simulink subsystem "PvtSubSys_LSM"  (R2020b)
settings: Solver=VariableStepAuto  StartTime=0.0  StopTime=10.0  RelTol=1e-3
values from neighbouring files (symbols this model uses):
  P_LSM_ALC_Enable = 0.0    [LSM_Parameter.sldd]
  P_LSM_DOP_C0_EN_Limit = 0.8    [LSM_Parameter.sldd]
  P_LSM_DOP_C0_out_Limit = 2.0    [LSM_Parameter.sldd]
  P_LSM_DOP_C1_EN_Limit : value not decoded    [LSM_Parameter.sldd]
  P_LSM_DOP_C1_out_Limit : value not decoded    [LSM_Parameter.sldd]
  P_LSM_DOP_C1AndC2_Lim_X : value not decoded    [LSM_Parameter.sldd]
  P_LSM_DOP_C2_EN_Limit : value not decoded    [LSM_Parameter.sldd]
  P_LSM_DOP_C2_out_Limit : value not decoded    [LSM_Parameter.sldd]
  P_LSM_DOP_In_Pre2Dop_Dis = 1.0    [LSM_Parameter.sldd]
  P_LSM_DOP_Out_Pre2Dop_Dis = 2.0    [LSM_Parameter.sldd]
  P_LSM_DOP_PreDis_X : value not decoded    [LSM_Parameter.sldd]
  P_LSM_DOP_PreDis_Y : value not decoded    [LSM_Parameter.sldd]
  P_LSM_DOPValid_CheckTime = 0.06    [LSM_Parameter.sldd]
  P_LSM_DoubleLine_Curr2Cent_Dislimit = 0.5    [LSM_Parameter.sldd]
  P_LSM_DoubleLine_Dop2Cent_Dislimit = 0.5    [LSM_Parameter.sldd]
  P_LSM_DoubleLine_DOPOut_C1 : value not decoded    [LSM_Parameter.sldd]
  P_LSM_DoubleLine_Pre2Cent_Dislimit = 1.0    [LSM_Parameter.sldd]
  P_LSM_IFV2CenterAxis = 0.0    [LSM_Parameter.sldd]
  P_LSM_IFV2RearAxis = 0.0    [LSM_Parameter.sldd]
  P_LSM_LineSTD_Limit = 0.15    [LSM_Parameter.sldd]
  P_LSM_NOH_Switch = 0.0    [LSM_Parameter.sldd]
  P_LSM_Pre_t = 0.0    [LSM_Parameter.sldd]
  P_LSM_SingleLine_Cent2Edge_Dislimit = 100.0    [LSM_Parameter.sldd]
  P_LSM_SingleLine_Curr2Cent_Dislimit = 0.2    [LSM_Parameter.sldd]
  P_LSM_SingleLine_Dop2Cent_Dislimit = 0.2    [LSM_Parameter.sldd]
  P_LSM_SingleLine_DOPOut_C1 : value not decoded    [LSM_Parameter.sldd]
  P_LSM_SingleLine_Pre2Cent_Dislimit = 0.5    [LSM_Parameter.sldd]
undefined symbols (not defined in the file or in its folder): P_LSM_LineWijCal_C12, P_LSM_LineWijCal_C13, P_LSM_PosLineLcFac
libraries: simulink x92, TrueDurationTime x2
(part 5 of 9)

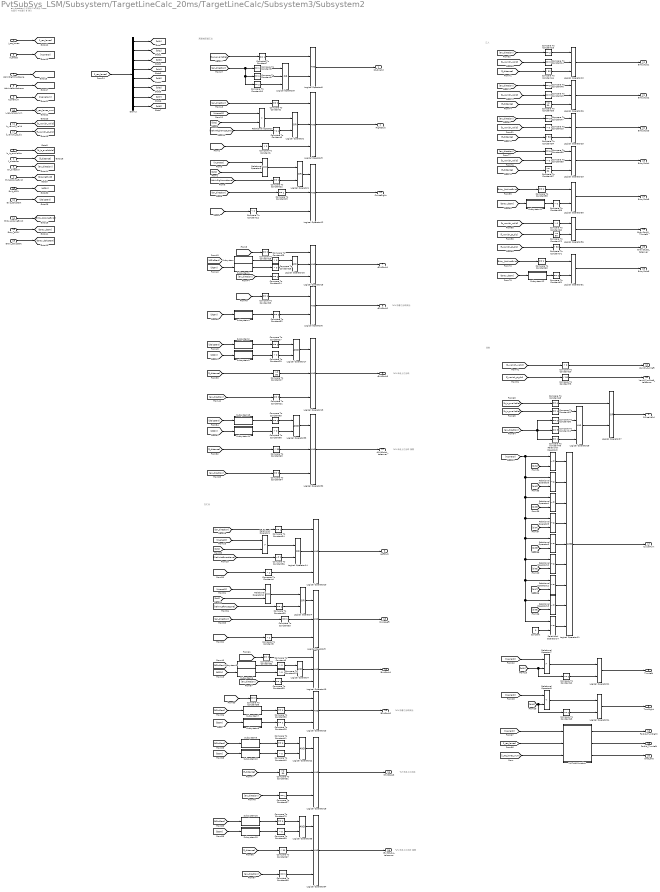
== system PvtSubSys_LSM/Subsystem/TargetLineCalc_20ms/TargetLineCalc/Subsystem3/Subsystem2 ==
  note: 左汇出
  note: 巡航
  note: 汇入
  note: %%未走上汇出线
  note: %%沿着汇出线驶出
  note: %%未走上汇出线
  note: en_direction
      | 1 左驶出
      | 2 右驶出
      | 3 左直行
      | 4 右直行
      | 5 驶入
  note: %%沿着汇出线驶出
  note: 高速或匝道汇出
  note: %%未走上汇出线,接管
  note: %%未走上汇出线,接管
  Exit_bIsLineExist : Inport
  f_distance : Inport  Port=2
  b_is_available : Inport  Port=3
  i_rec_lanes : Inport  Port=4
  nLaneID : Inport  Port=5
  en_direction : Inport  Port=6
  VehInRightmostLane : Inport  Port=7  OutDataTypeStr=boolean
  VehInLeftmostLane : Inport  Port=8  OutDataTypeStr=boolean
  nLaneNum : Inport  Port=9
  i_rec_lanes_num : Inport  Port=10
  " b_vanish_valid" : Inport  Port=11
  " Exit_dDisStart" : Inport  Port=12
  Exit_dC0V : Inport  Port=13
  Entry_bIsLineExist : Inport  Port=14
  Entry_dDisStart : Inport  Port=15
  Entry_dC0V : Inport  Port=16
  " f_vanish_pt_dis " : Inport  Port=17
  Compare To Constant{1,4..5,12} (4 alike) : simulink/Logic and Bit Operations/Compare To Constant  relop=<  const=2  OutDataTypeStr=boolean
  Compare To Constant{10,16,46..47,56} (5 alike) : simulink/Logic and Bit Operations/Compare To Constant  relop===  const=5  OutDataTypeStr=boolean
  Compare To Constant11 : simulink/Logic and Bit Operations/Compare To Constant  relop===  const=3  OutDataTypeStr=boolean
  Compare To Constant{6,13,15,20,25..26,29,40,55,59,62,66,69} (13 alike) : simulink/Logic and Bit Operations/Compare To Constant  relop=>  const=0  OutDataTypeStr=boolean
  Compare To Constant{14,27..28,30,41,45,48,50,52,61,65,70} (12 alike) : simulink/Logic and Bit Operations/Compare To Constant  relop===  const=0  OutDataTypeStr=boolean
  Compare To Constant17 : simulink/Logic and Bit Operations/Compare To Constant  relop=>=  const=50  OutDataTypeStr=boolean
  Compare To Constant{2,9,18..19,21,23..24,32,38,58,60,64} (12 alike) : simulink/Logic and Bit Operations/Compare To Constant  relop===  const=2  OutDataTypeStr=boolean
  Compare To Constant{7..8,22,33..35,37,39,51,68} (10 alike) : simulink/Logic and Bit Operations/Compare To Constant  relop===  const=1  OutDataTypeStr=boolean
  Compare To Constant3 : simulink/Logic and Bit Operations/Compare To Constant  relop=~=  const=1  OutDataTypeStr=boolean
  Compare To Constant31 : simulink/Logic and Bit Operations/Compare To Constant  relop=>=  const=50  OutDataTypeStr=boolean
  Compare To Constant36 : simulink/Logic and Bit Operations/Compare To Constant  relop=~=  const=1  OutDataTypeStr=boolean
  Compare To Constant42 : simulink/Logic and Bit Operations/Compare To Constant  relop=~=  const=0  OutDataTypeStr=boolean
  Compare To Constant43 : simulink/Logic and Bit Operations/Compare To Constant  relop=~=  const=0  OutDataTypeStr=boolean
  Compare To Constant44 : simulink/Logic and Bit Operations/Compare To Constant  relop=>  const=50  OutDataTypeStr=boolean
  Compare To Constant49 : simulink/Logic and Bit Operations/Compare To Constant  relop===  const=4  OutDataTypeStr=boolean
  Compare To Constant53 : simulink/Logic and Bit Operations/Compare To Constant  relop=<=  const=50  OutDataTypeStr=boolean
  Compare To Constant54 : simulink/Logic and Bit Operations/Compare To Constant  relop=>  const=50  OutDataTypeStr=boolean
  Compare To Constant57 : simulink/Logic and Bit Operations/Compare To Constant  relop=<=  const=50  OutDataTypeStr=boolean
  Compare To Constant{63,67,71,73} (4 alike) : simulink/Logic and Bit Operations/Compare To Constant  relop=<  const=50  OutDataTypeStr=boolean
  Compare To Constant72 : simulink/Logic and Bit Operations/Compare To Constant  relop=>=  const=50  OutDataTypeStr=boolean
  Constant : Constant  Value=0  OutDataTypeStr=uint8
  Demux : Demux  Outputs=8
  Logical Operator{1..2,4,14,27} (5 alike) : Logic  Operator=OR  AllPortsSameDT=off  OutDataTypeStr=boolean
  Logical Operator{3,5,10,12..13,15,18..20,23,25..26,29,32,34} (15 alike) : Logic  Inputs=3  AllPortsSameDT=off  OutDataTypeStr=boolean
  Logical Operator11 : Logic  Inputs=9'  AllPortsSameDT=off  OutDataTypeStr=boolean
  Logical Operator{6..8,16..17,21..22,24,30..31,33,35..36} (13 alike) : Logic  AllPortsSameDT=off  OutDataTypeStr=boolean
  Logical Operator28 : Logic  Inputs=4  AllPortsSameDT=off  OutDataTypeStr=boolean
  Logical Operator9 : Logic  Operator=OR  Inputs=3  AllPortsSameDT=off  OutDataTypeStr=boolean
  MATLAB Function : MATLAB Function  TreatAsAtomicUnit=on
  Relational Operator : RelationalOperator  Operator=<  OutDataTypeStr=boolean  RndMeth=Simplest
  Relational Operator1 : RelationalOperator  Operator=>  OutDataTypeStr=boolean  RndMeth=Simplest
  Relational Operator{2..6,10,12..14} (9 alike) : RelationalOperator  Operator=~=  OutDataTypeStr=boolean  RndMeth=Simplest
  Relational Operator11 : RelationalOperator  Operator===  OutDataTypeStr=boolean  RndMeth=Simplest
  Relational Operator7 : RelationalOperator  Operator=>  OutDataTypeStr=boolean  RndMeth=Simplest
  Relational Operator8 : RelationalOperator  Operator=<  OutDataTypeStr=boolean  RndMeth=Simplest
  Relational Operator9 : RelationalOperator  Operator===  OutDataTypeStr=boolean  RndMeth=Simplest
  Subsystem : Subsystem
  Subsystem1 : Subsystem
  Subsystem10 : Subsystem
  Subsystem11 : Subsystem
  Subsystem12 : Subsystem
  Subsystem13 : Subsystem
  Subsystem14 : Subsystem
  Subsystem15 : Subsystem
  Subsystem16 : Subsystem
  Subsystem2 : Subsystem
  Subsystem3 : Subsystem
  Subsystem4 : Subsystem
  Subsystem5 : Subsystem
  Subsystem6 : Subsystem
  Subsystem7 : Subsystem
  Subsystem8 : Subsystem
  Subsystem9 : Subsystem
  StubValid : Outport
  RightStub : Outport  Port=2
  LeftStub : Outport  Port=3
  CruiseValid : Outport  Port=4
  TurnLeft : Outport  Port=5
  TurnRight : Outport  Port=6
  rExitStub1 : Outport  Port=7
  rExitStub2 : Outport  Port=8
  rExitStub3 : Outport  Port=9
  Vanish_turnleft : Outport  Port=10
  EntryStub1 : Outport  Port=11
  CruiseRight : Outport  Port=12
  CruiseLeft : Outport  Port=13
  lExitStub1 : Outport  Port=14
  lExitStub2 : Outport  Port=15
  lExitStub3 : Outport  Port=16
  CruiseTurn : Outport  Port=17
  Forbid_TurnRight : Outport  Port=18
  Forbid_TurnLeft : Outport  Port=19
  OneLane : Outport  Port=20
  EntryStub2 : Outport  Port=21
  EntryStub3 : Outport  Port=22
  EntryStub4 : Outport  Port=23
  EntryStub5 : Outport  Port=24
  EntryStub6 : Outport  Port=25
  EntryStub5_TurnLeft : Outport  Port=26
  rExitStub4_takeover : Outport  Port=27
  lExitStub4_takeover : Outport  Port=28
  EntryStub5_takeover : Outport  Port=29
  Vanish_turnleft_takeover : Outport  Port=30
  wires:
  Compare To Constant40/1 -> Logical Operator22/2
  Compare To Constant41/1 -> Logical Operator22/1
  Subsystem9/1(y) -> Compare To Constant41/1
  [dDisStart] -> Subsystem9/1(u)
  [dC0V] -> Subsystem10/1(u)
  Subsystem10/1(y) -> Compare To Constant40/1
  Subsystem8/1(y) -> Compare To Constant28/1
  [dC0V] -> Subsystem8/1(u)
  [dDisStart] -> Subsystem7/1(u)
  Subsystem7/1(y) -> Compare To Constant30/1
  Compare To Constant30/1 -> Logical Operator23/2
  Compare To Constant28/1 -> Logical Operator23/3
  Logical Operator7/1 -> Logical Operator19/2
  Compare To Constant13/1 -> Logical Operator7/2
  Compare To Constant6/1 -> Logical Operator7/1
  Subsystem5/1(y) -> Compare To Constant6/1
  [dDisStart] -> Subsystem5/1(u)
  [dC0V] -> Subsystem6/1(u)
  Subsystem6/1(y) -> Compare To Constant13/1
  Subsystem3/1(y) -> Compare To Constant29/1
  [dC0V] -> Subsystem3/1(u)
  [dDisStart] -> Subsystem2/1(u)
  Subsystem2/1(y) -> Compare To Constant27/1
  Compare To Constant27/1 -> Logical Operator17/1
  Compare To Constant29/1 -> Logical Operator17/2
  Compare To Constant52/1 -> Logical Operator6/2
  [dC0V] -> Subsystem4/1(u)
  Subsystem4/1(y) -> Compare To Constant52/1
  Subsystem1/1(y) -> Compare To Constant26/1
  [dC0V] -> Subsystem1/1(u)
  [dDisStart] -> Subsystem/1(u)
  [i_rec_lanes_num] -> MATLAB Function/3(i_rec_lanes_num)
  MATLAB Function/3(OneLane) -> OneLane/1
  MATLAB Function/2(Forbid_TurnLeft) -> Forbid_TurnLeft/1
  MATLAB Function/1(Forbid_TurnRight) -> Forbid_TurnRight/1
  [nLaneID] -> MATLAB Function/1(nLaneID)
  [i_rec_lanes] -> MATLAB Function/2(i_rec_lanes)
  Logical Operator27/1 -> CruiseValid/1  "CruiseValid"
  Compare To Constant49/1 -> Logical Operator28/4
  Compare To Constant51/1 -> Logical Operator28/1
  [b_is_available] -> Compare To Constant51/1
  [en_direction] -> Compare To Constant11/1, Compare To Constant49/1, Compare To Constant50/1
  Compare To Constant50/1 -> Logical Operator28/2
  Compare To Constant11/1 -> Logical Operator28/3
  Logical Operator28/1 -> Logical Operator27/2
  Constant/1 -> Relational Operator14/2
  Relational Operator14/1 -> Logical Operator11/9
  Compare To Constant12/1 -> Logical Operator12/3
  Logical Operator8/1 -> StubValid/1  "StubValid"
  Logical Operator9/1 -> Logical Operator8/2
  Compare To Constant10/1 -> Logical Operator9/3
  Compare To Constant9/1 -> Logical Operator9/2
  Compare To Constant8/1 -> Logical Operator9/1
  [en_direction] -> Compare To Constant8/1, Compare To Constant9/1, Compare To Constant10/1
  Relational Operator7/1 -> Logical Operator21/1
  [bit8] -> Relational Operator13/2
  [bit7] -> Relational Operator12/2
  [bit6] -> Relational Operator10/2
  Relational Operator13/1 -> Logical Operator11/8
  Relational Operator12/1 -> Logical Operator11/7
  Relational Operator10/1 -> Logical Operator11/6
  [b_is_available] -> Compare To Constant48/1
  Compare To Constant48/1 -> Logical Operator27/1
  Compare To Constant37/1 -> Logical Operator18/3
  Logical Operator19/1 -> lExitStub1/1  "lExitStub1"
  [en_direction] -> Compare To Constant37/1
  Compare To Constant39/1 -> Logical Operator19/3
  [f_distance] -> Compare To Constant31/1
  [en_direction] -> Compare To Constant39/1
  Logical Operator18/1 -> lExitStub3/1  "lExitStub3"
  Logical Operator22/1 -> Logical Operator18/1
  Compare To Constant31/1 -> Logical Operator18/2
  [bIsLineExist] -> Compare To Constant32/1
  Compare To Constant32/1 -> Logical Operator19/1
  Compare To Constant38/1 -> Logical Operator23/1
  [bIsLineExist] -> Compare To Constant38/1
  Logical Operator23/1 -> lExitStub2/1  "lExitStub2"
  Logical Operator20/1 -> LeftStub/1  "LeftStub"
  [en_direction] -> Compare To Constant33/1  "LSM_Stub_Direction"
  Relational Operator1/1 -> Logical Operator14/1
  [bit1] -> Relational Operator1/2
  Logical Operator5/1 -> CruiseLeft/1  "CruiseLeft"
  [VehInLeftmostLane] -> Compare To Constant36/1
  Relational Operator11/1 -> Logical Operator4/1
  [nLaneID] -> Relational Operator1/1
  [VehInLeftmostLane] -> Compare To Constant35/1
  Compare To Constant35/1 -> Logical Operator4/2
  Logical Operator4/1 -> Logical Operator5/1
  Compare To Constant33/1 -> Logical Operator5/2
  [en_direction] -> Compare To Constant34/1  "LSM_Stub_Direction"
  Compare To Constant34/1 -> Logical Operator20/1
  [nLaneID] -> Relational Operator11/1
  [bit1] -> Relational Operator11/2
  Compare To Constant5/1 -> Logical Operator5/3
  Logical Operator14/1 -> Logical Operator20/2
  [bIsLineExist] -> Compare To Constant5/1
  Compare To Constant4/1 -> Logical Operator20/3
  [bIsLineExist] -> Compare To Constant4/1
  Compare To Constant36/1 -> Logical Operator14/2
  Logical Operator6/1 -> rExitStub2/1  "rExitStub2"
  [bIsLineExist] -> Compare To Constant23/1
  Compare To Constant23/1 -> Logical Operator6/1
  Compare To Constant18/1 -> Logical Operator15/1
  [bIsLineExist] -> Compare To Constant18/1
  [bIsLineExist] -> Compare To Constant12/1
  Exit_bIsLineExist/1 -> [bIsLineExist]
  Compare To Constant1/1 -> Logical Operator3/3
  [bIsLineExist] -> Compare To Constant1/1
  [b_is_available] -> Compare To Constant7/1
  b_is_available/1 -> [b_is_available]
  Compare To Constant22/1 -> Logical Operator1/2
  [en_direction] -> Compare To Constant19/1  "LSM_Stub_Direction"
  [bit1] -> Relational Operator9/2
  Compare To Constant19/1 -> Logical Operator12/2
  Relational Operator9/1 -> Logical Operator1/1
  Logical Operator1/1 -> Logical Operator12/1
  Logical Operator12/1 -> CruiseRight/1  "CruiseRight"
  [VehInRightmostLane] -> Compare To Constant22/1
  [nLaneID] -> Relational Operator9/1
  Logical Operator10/1 -> EntryStub1/1  "EntryStub1"
  Logical Operator11/1 -> CruiseTurn/1  "CruiseTurn"
  Compare To Constant17/1 -> Logical Operator13/2
  VehInRightmostLane/1 -> [VehInRightmostLane]
  " Exit_dDisStart"/1 -> [dDisStart]
  nLaneID/1 -> [nLaneID]
  VehInLeftmostLane/1 -> [VehInLeftmostLane]
  f_distance/1 -> [f_distance]
  [en_direction] -> Compare To Constant2/1  "LSM_Stub_Direction"
  Relational Operator2/1 -> Logical Operator11/1
  Relational Operator4/1 -> Logical Operator11/3
  [bit1] -> Relational Operator2/2
  [bit1] -> Compare To Constant43/1, Relational Operator8/2
  [nLaneID] -> Relational Operator8/1
  Relational Operator8/1 -> Logical Operator24/1
  [nLaneID] -> Relational Operator/1
  [bit1] -> Compare To Constant42/1, Relational Operator7/2
  [en_direction] -> Compare To Constant16/1  "LSM_Stub_Direction"
  Logical Operator17/1 -> Logical Operator13/1
  nLaneNum/1 -> [nLaneNum]
  i_rec_lanes_num/1 -> [i_rec_lanes_num]
  [b_vanish_valid] -> Compare To Constant14/1
  Compare To Constant20/1 -> Vanish_turnleft/1  "Vanish_turnleft"
  Subsystem/1(y) -> Compare To Constant25/1
  Logical Operator3/1 -> RightStub/1  "RightStub"
  Logical Operator16/1 -> Logical Operator15/2
  [bit1] -> Relational Operator/2
  [bit2] -> Relational Operator3/2
  [bit3] -> Relational Operator4/2
  Compare To Constant14/1 -> Logical Operator10/2
  [bit5] -> Relational Operator6/2
  Exit_dC0V/1 -> [dC0V]
  [VehInRightmostLane] -> Compare To Constant3/1
  Compare To Constant7/1 -> Logical Operator8/1
  Logical Operator13/1 -> rExitStub3/1  "rExitStub3"
  " b_vanish_valid"/1 -> [b_vanish_valid]
  [en_direction] -> Compare To Constant24/1
  [bit4] -> Relational Operator5/2
  Compare To Constant2/1 -> Logical Operator3/1
  Logical Operator2/1 -> Logical Operator3/2
  Relational Operator/1 -> Logical Operator2/1
  Compare To Constant16/1 -> Logical Operator10/1
  [b_vanish_valid] -> Compare To Constant20/1
  [f_distance] -> Compare To Constant17/1
  Relational Operator6/1 -> Logical Operator11/5
  [nLaneID] -> Relational Operator2/1, Relational Operator6/1, Relational Operator13/1, Relational Operator14/1, Relational Operator12/1, Relational Operator10/1, Relational Operator5/1, Relational Operator4/1, Relational Operator3/1
  en_direction/1 -> [en_direction]
  Compare To Constant24/1 -> Logical Operator15/3
  Compare To Constant25/1 -> Logical Operator16/1
  [en_direction] -> Compare To Constant21/1
  Logical Operator15/1 -> rExitStub1/1  "rExitStub1"
  Relational Operator3/1 -> Logical Operator11/2
  Compare To Constant26/1 -> Logical Operator16/2
  Relational Operator5/1 -> Logical Operator11/4
  [nLaneID] -> Relational Operator7/1
  Compare To Constant3/1 -> Logical Operator2/2
  Compare To Constant21/1 -> Logical Operator13/3
  Compare To Constant42/1 -> Logical Operator21/2
  Logical Operator21/1 -> TurnLeft/1  "TurnLeft"
  Compare To Constant43/1 -> Logical Operator24/2
  Logical Operator24/1 -> TurnRight/1  "TurnLeft"
  [i_rec_lanes] -> Demux/1
  Demux/5 -> [bit5]
  Demux/4 -> [bit4]
  Demux/6 -> [bit6]
  Demux/7 -> [bit7]
  Demux/8 -> [bit8]
  Demux/1 -> [bit1]
  Demux/3 -> [bit3]
  Demux/2 -> [bit2]
  i_rec_lanes/1 -> [i_rec_lanes]
  Entry_dC0V/1 -> [Entry_dC0V]
  Entry_dDisStart/1 -> [Entry_dDisStart]
  Entry_bIsLineExist/1 -> [Entry_bIsLineExist]
  [f_distance] -> Compare To Constant44/1
  Compare To Constant44/1 -> Logical Operator10/3
  Compare To Constant53/1 -> Logical Operator26/3
  [f_distance] -> Compare To Constant53/1
  Compare To Constant46/1 -> Logical Operator26/1
  Compare To Constant45/1 -> Logical Operator26/2
  [b_vanish_valid] -> Compare To Constant45/1
  [en_direction] -> Compare To Constant46/1  "LSM_Stub_Direction"
  Logical Operator26/1 -> EntryStub2/1  "EntryStub2"
  Logical Operator29/1 -> EntryStub4/1  "EntryStub4"
  [en_direction] -> Compare To Constant56/1  "LSM_Stub_Direction"
  [b_vanish_valid] -> Compare To Constant55/1
  Compare To Constant55/1 -> Logical Operator29/2
  Compare To Constant56/1 -> Logical Operator29/1
  [f_distance] -> Compare To Constant57/1
  Compare To Constant57/1 -> Logical Operator29/3
  Compare To Constant54/1 -> Logical Operator25/3
  [f_distance] -> Compare To Constant54/1
  Compare To Constant47/1 -> Logical Operator25/1
  Compare To Constant15/1 -> Logical Operator25/2
  [b_vanish_valid] -> Compare To Constant15/1
  [en_direction] -> Compare To Constant47/1  "LSM_Stub_Direction"
  Logical Operator25/1 -> EntryStub3/1  "EntryStub3"
  [Entry_bIsLineExist] -> Compare To Constant58/1
  Compare To Constant58/1 -> Logical Operator30/1
  [Entry_dC0V] -> Subsystem11/1(u)
  Subsystem11/1(y) -> Compare To Constant59/1
  Compare To Constant59/1 -> Logical Operator30/2
  Logical Operator30/1 -> EntryStub5/1  "EntryStub5"
  Logical Operator31/1 -> EntryStub6/1  "EntryStub6"
  Compare To Constant61/1 -> Logical Operator31/2
  Subsystem12/1(y) -> Compare To Constant61/1
  [Entry_dC0V] -> Subsystem12/1(u)
  Compare To Constant60/1 -> Logical Operator31/1
  [Entry_bIsLineExist] -> Compare To Constant60/1
  Compare To Constant62/1 -> Logical Operator36/1
  [b_vanish_valid] -> Compare To Constant62/1
  Compare To Constant64/1 -> Logical Operator32/3
  [en_direction] -> Compare To Constant64/1
  [f_distance] -> Compare To Constant63/1
  Logical Operator32/1 -> rExitStub4_takeover/1  "rExitStub4_takeover"
  Logical Operator33/1 -> Logical Operator32/1
  Compare To Constant63/1 -> Logical Operator32/2
  Compare To Constant66/1 -> Logical Operator33/2
  Compare To Constant65/1 -> Logical Operator33/1
  Subsystem13/1(y) -> Compare To Constant65/1
  [dDisStart] -> Subsystem13/1(u)
  [dC0V] -> Subsystem14/1(u)
  Subsystem14/1(y) -> Compare To Constant66/1
  Compare To Constant67/1 -> Logical Operator34/2
  Logical Operator35/1 -> Logical Operator34/1
  Logical Operator34/1 -> lExitStub4_takeover/1  "lExitStub4_takeover"
  [f_distance] -> Compare To Constant67/1
  [en_direction] -> Compare To Constant68/1
  Compare To Constant68/1 -> Logical Operator34/3
  Subsystem15/1(y) -> Compare To Constant69/1
  [dC0V] -> Subsystem15/1(u)
  [dDisStart] -> Subsystem16/1(u)
  Subsystem16/1(y) -> Compare To Constant70/1
  Compare To Constant70/1 -> Logical Operator35/1
  Compare To Constant69/1 -> Logical Operator35/2
  [f_vanish_pt_dis] -> Compare To Constant71/1
  Compare To Constant71/1 -> EntryStub5_takeover/1  "EntryStub5_takeover"
  " f_vanish_pt_dis "/1 -> [f_vanish_pt_dis]
  [f_vanish_pt_dis] -> Compare To Constant72/1
  Compare To Constant72/1 -> Logical Operator36/2
  Logical Operator36/1 -> EntryStub5_TurnLeft/1  "EntryStub5_TurnLeft"
  [f_vanish_pt_dis] -> Compare To Constant73/1
  Compare To Constant73/1 -> Vanish_turnleft_takeover/1  "Vanish_turnleft_takeover"

== system PvtSubSys_LSM/Subsystem/TargetLineCalc_20ms/TargetLineCalc/Subsystem3/Subsystem3 ==
  PilotTurnSwSts : Inport
  nLaneID : Inport  Port=2
  Compare To Constant2 : simulink/Logic and Bit Operations/Compare To Constant  relop===  const=1  OutDataTypeStr=boolean
  Compare To Constant3 : simulink/Logic and Bit Operations/Compare To Constant  relop===  const=2  OutDataTypeStr=boolean
  Constant : Constant  OutDataTypeStr=uint8
  Constant1 : Constant  Value=2  OutDataTypeStr=uint8
  Constant2 : Constant  Value=0  OutDataTypeStr=uint8
  Logical Operator1 : Logic  AllPortsSameDT=off  OutDataTypeStr=boolean
  Logical Operator2 : Logic  AllPortsSameDT=off  OutDataTypeStr=boolean
  Relational Operator1 : RelationalOperator  Operator=<  OutDataTypeStr=boolean  RndMeth=Simplest
  Relational Operator2 : RelationalOperator  Operator=>  OutDataTypeStr=boolean  RndMeth=Simplest
  Switch : Switch  Criteria=u2 > Threshold
  Switch1 : Switch  Criteria=u2 > Threshold
  Unit Delay{,1..3} (4 alike) : UnitDelay  SampleTime=-1  HasFrameUpgradeWarning=on
  LaneChange : Outport
  wires:
  Relational Operator1/1 -> Logical Operator1/2
  Compare To Constant2/1 -> Logical Operator1/1
  Constant/1 -> Switch/1
  Constant2/1 -> Switch1/3
  Unit Delay2/1 -> Compare To Constant3/1
  Logical Operator1/1 -> Switch/2
  Unit Delay/1 -> Relational Operator1/2
  PilotTurnSwSts/1 -> Unit Delay2/1, Unit Delay3/1
  Logical Operator2/1 -> Switch1/2
  Unit Delay3/1 -> Compare To Constant2/1
  Constant1/1 -> Switch1/1
  Unit Delay1/1 -> Relational Operator2/2
  Compare To Constant3/1 -> Logical Operator2/1
  Switch1/1 -> Switch/3
  nLaneID/1 -> Relational Operator2/1, Unit Delay1/1, Unit Delay/1, Relational Operator1/1
  Relational Operator2/1 -> Logical Operator2/2
  Switch/1 -> LaneChange/1  "LaneChange"

== system PvtSubSys_LSM/Subsystem/TargetLineCalc_20ms/TargetLineCalc/Subsystem4/If Action Subsystem ==
  In1 : Inport
  Action Port : ActionPort
  LH1Wij : Outport
  wires:
  In1/1 -> LH1Wij/1

== system PvtSubSys_LSM/Subsystem/TargetLineCalc_20ms/TargetLineCalc/Subsystem4/If Action Subsystem1 ==
  In1 : Inport
  Action Port : ActionPort
  LH1Wij : Outport
  wires:
  In1/1 -> LH1Wij/1

== system PvtSubSys_LSM/Subsystem/TargetLineCalc_20ms/TargetLineCalc/Subsystem4/If Action Subsystem2 ==
  Action Port : ActionPort
  Constant : Constant  Value=0  OutDataTypeStr=single
  LH1Wij : Outport
  wires:
  Constant/1 -> LH1Wij/1

== system PvtSubSys_LSM/Subsystem/TargetLineCalc_20ms/TargetLineCalc/Subsystem4/If Action Subsystem3 ==
  Action Port : ActionPort
  Constant : Constant  Value=0  OutDataTypeStr=single
  LH1Wij : Outport
  wires:
  Constant/1 -> LH1Wij/1

== system PvtSubSys_LSM/Subsystem/TargetLineCalc_20ms/TargetLineCalc/Subsystem4/If Action Subsystem4 ==
  In1 : Inport
  In2 : Inport  Port=2
  Action Port : ActionPort
  Out1 : Outport
  Out2 : Outport  Port=2
  wires:
  In1/1 -> Out1/1
  In2/1 -> Out2/1

== system PvtSubSys_LSM/Subsystem/TargetLineCalc_20ms/TargetLineCalc/Subsystem4/If Action Subsystem5 ==
  Action Port : ActionPort
  Constant : Constant  Value=P_LSM_PosLineLcFac
  Out1 : Outport
  Out2 : Outport  Port=2
  wires:
  Constant/1 -> Out2/1, Out1/1

== system PvtSubSys_LSM/Subsystem/TargetLineCalc_20ms/TargetLineCalc/Subsystem5/If Action Subsystem ==
  In1 : Inport
  Action Port : ActionPort
  LH1Wij : Outport
  wires:
  In1/1 -> LH1Wij/1

== system PvtSubSys_LSM/Subsystem/TargetLineCalc_20ms/TargetLineCalc/Subsystem5/If Action Subsystem1 ==
  In1 : Inport
  Action Port : ActionPort
  LH1Wij : Outport
  wires:
  In1/1 -> LH1Wij/1

== system PvtSubSys_LSM/Subsystem/TargetLineCalc_20ms/TargetLineCalc/Subsystem5/If Action Subsystem2 ==
  Action Port : ActionPort
  Constant : Constant  Value=0  OutDataTypeStr=single
  LH1Wij : Outport
  wires:
  Constant/1 -> LH1Wij/1

== system PvtSubSys_LSM/Subsystem/TargetLineCalc_20ms/TargetLineCalc/Subsystem5/If Action Subsystem3 ==
  Action Port : ActionPort
  Constant : Constant  Value=0  OutDataTypeStr=single
  LH1Wij : Outport
  wires:
  Constant/1 -> LH1Wij/1

== system PvtSubSys_LSM/Subsystem/TargetLineCalc_20ms/TargetLineCalc/Subsystem5/If Action Subsystem4 ==
  In1 : Inport
  In2 : Inport  Port=2
  Action Port : ActionPort
  Out1 : Outport
  Out2 : Outport  Port=2
  wires:
  In1/1 -> Out1/1
  In2/1 -> Out2/1

== system PvtSubSys_LSM/Subsystem/TargetLineCalc_20ms/TargetLineCalc/Subsystem5/If Action Subsystem5 ==
  Action Port : ActionPort
  Constant : Constant  Value=P_LSM_PosLineLcFac
  Out1 : Outport
  Out2 : Outport  Port=2
  wires:
  Constant/1 -> Out2/1, Out1/1

== system PvtSubSys_LSM/Subsystem/TargetLineCalc_20ms/TargetLineCalc/Subsystem3/Subsystem2/Subsystem ==
  u : Inport
  MATLAB Function14 : MATLAB Function  TreatAsAtomicUnit=on
  Unit Delay : UnitDelay  SampleTime=-1  HasFrameUpgradeWarning=on
  y : Outport
  wires:
  MATLAB Function14/1(y) -> y/1
  Unit Delay/1 -> MATLAB Function14/2(i_k)
  u/1 -> MATLAB Function14/1(u)
  MATLAB Function14/2(i) -> Unit Delay/1

== system PvtSubSys_LSM/Subsystem/TargetLineCalc_20ms/TargetLineCalc/Subsystem3/Subsystem2/Subsystem1 ==
  u : Inport
  MATLAB Function14 : MATLAB Function  TreatAsAtomicUnit=on
  Unit Delay : UnitDelay  SampleTime=-1  HasFrameUpgradeWarning=on
  y : Outport
  wires:
  MATLAB Function14/2(i) -> Unit Delay/1
  u/1 -> MATLAB Function14/1(u)
  Unit Delay/1 -> MATLAB Function14/2(i_k)
  MATLAB Function14/1(y) -> y/1

== system PvtSubSys_LSM/Subsystem/TargetLineCalc_20ms/TargetLineCalc/Subsystem3/Subsystem2/Subsystem10 ==
  u : Inport
  MATLAB Function14 : MATLAB Function  TreatAsAtomicUnit=on
  Unit Delay : UnitDelay  SampleTime=-1  HasFrameUpgradeWarning=on
  y : Outport
  wires:
  MATLAB Function14/2(i) -> Unit Delay/1
  u/1 -> MATLAB Function14/1(u)
  Unit Delay/1 -> MATLAB Function14/2(i_k)
  MATLAB Function14/1(y) -> y/1

== system PvtSubSys_LSM/Subsystem/TargetLineCalc_20ms/TargetLineCalc/Subsystem3/Subsystem2/Subsystem11 ==
  u : Inport
  MATLAB Function14 : MATLAB Function  TreatAsAtomicUnit=on
  Unit Delay : UnitDelay  SampleTime=-1  HasFrameUpgradeWarning=on
  y : Outport
  wires:
  MATLAB Function14/1(y) -> y/1
  Unit Delay/1 -> MATLAB Function14/2(i_k)
  u/1 -> MATLAB Function14/1(u)
  MATLAB Function14/2(i) -> Unit Delay/1

== system PvtSubSys_LSM/Subsystem/TargetLineCalc_20ms/TargetLineCalc/Subsystem3/Subsystem2/Subsystem12 ==
  u : Inport
  MATLAB Function14 : MATLAB Function  TreatAsAtomicUnit=on
  Unit Delay : UnitDelay  SampleTime=-1  HasFrameUpgradeWarning=on
  y : Outport
  wires:
  MATLAB Function14/2(i) -> Unit Delay/1
  u/1 -> MATLAB Function14/1(u)
  Unit Delay/1 -> MATLAB Function14/2(i_k)
  MATLAB Function14/1(y) -> y/1

== system PvtSubSys_LSM/Subsystem/TargetLineCalc_20ms/TargetLineCalc/Subsystem3/Subsystem2/Subsystem13 ==
  u : Inport
  MATLAB Function14 : MATLAB Function  TreatAsAtomicUnit=on
  Unit Delay : UnitDelay  SampleTime=-1  HasFrameUpgradeWarning=on
  y : Outport
  wires:
  MATLAB Function14/2(i) -> Unit Delay/1
  u/1 -> MATLAB Function14/1(u)
  Unit Delay/1 -> MATLAB Function14/2(i_k)
  MATLAB Function14/1(y) -> y/1

== system PvtSubSys_LSM/Subsystem/TargetLineCalc_20ms/TargetLineCalc/Subsystem3/Subsystem2/Subsystem14 ==
  u : Inport
  MATLAB Function14 : MATLAB Function  TreatAsAtomicUnit=on
  Unit Delay : UnitDelay  SampleTime=-1  HasFrameUpgradeWarning=on
  y : Outport
  wires:
  MATLAB Function14/1(y) -> y/1
  Unit Delay/1 -> MATLAB Function14/2(i_k)
  u/1 -> MATLAB Function14/1(u)
  MATLAB Function14/2(i) -> Unit Delay/1

== system PvtSubSys_LSM/Subsystem/TargetLineCalc_20ms/TargetLineCalc/Subsystem3/Subsystem2/Subsystem15 ==
  u : Inport
  MATLAB Function14 : MATLAB Function  TreatAsAtomicUnit=on
  Unit Delay : UnitDelay  SampleTime=-1  HasFrameUpgradeWarning=on
  y : Outport
  wires:
  MATLAB Function14/1(y) -> y/1
  Unit Delay/1 -> MATLAB Function14/2(i_k)
  u/1 -> MATLAB Function14/1(u)
  MATLAB Function14/2(i) -> Unit Delay/1

== system PvtSubSys_LSM/Subsystem/TargetLineCalc_20ms/TargetLineCalc/Subsystem3/Subsystem2/Subsystem16 ==
  u : Inport
  MATLAB Function14 : MATLAB Function  TreatAsAtomicUnit=on
  Unit Delay : UnitDelay  SampleTime=-1  HasFrameUpgradeWarning=on
  y : Outport
  wires:
  MATLAB Function14/2(i) -> Unit Delay/1
  u/1 -> MATLAB Function14/1(u)
  Unit Delay/1 -> MATLAB Function14/2(i_k)
  MATLAB Function14/1(y) -> y/1

== system PvtSubSys_LSM/Subsystem/TargetLineCalc_20ms/TargetLineCalc/Subsystem3/Subsystem2/Subsystem2 ==
  u : Inport
  MATLAB Function14 : MATLAB Function  TreatAsAtomicUnit=on
  Unit Delay : UnitDelay  SampleTime=-1  HasFrameUpgradeWarning=on
  y : Outport
  wires:
  MATLAB Function14/1(y) -> y/1
  Unit Delay/1 -> MATLAB Function14/2(i_k)
  u/1 -> MATLAB Function14/1(u)
  MATLAB Function14/2(i) -> Unit Delay/1

== system PvtSubSys_LSM/Subsystem/TargetLineCalc_20ms/TargetLineCalc/Subsystem3/Subsystem2/Subsystem3 ==
  u : Inport
  MATLAB Function14 : MATLAB Function  TreatAsAtomicUnit=on
  Unit Delay : UnitDelay  SampleTime=-1  HasFrameUpgradeWarning=on
  y : Outport
  wires:
  MATLAB Function14/2(i) -> Unit Delay/1
  u/1 -> MATLAB Function14/1(u)
  Unit Delay/1 -> MATLAB Function14/2(i_k)
  MATLAB Function14/1(y) -> y/1

== system PvtSubSys_LSM/Subsystem/TargetLineCalc_20ms/TargetLineCalc/Subsystem3/Subsystem2/Subsystem4 ==
  u : Inport
  MATLAB Function14 : MATLAB Function  TreatAsAtomicUnit=on
  Unit Delay : UnitDelay  SampleTime=-1  HasFrameUpgradeWarning=on
  y : Outport
  wires:
  MATLAB Function14/1(y) -> y/1
  Unit Delay/1 -> MATLAB Function14/2(i_k)
  u/1 -> MATLAB Function14/1(u)
  MATLAB Function14/2(i) -> Unit Delay/1

== system PvtSubSys_LSM/Subsystem/TargetLineCalc_20ms/TargetLineCalc/Subsystem3/Subsystem2/Subsystem5 ==
  u : Inport
  MATLAB Function14 : MATLAB Function  TreatAsAtomicUnit=on
  Unit Delay : UnitDelay  SampleTime=-1  HasFrameUpgradeWarning=on
  y : Outport
  wires:
  MATLAB Function14/1(y) -> y/1
  Unit Delay/1 -> MATLAB Function14/2(i_k)
  u/1 -> MATLAB Function14/1(u)
  MATLAB Function14/2(i) -> Unit Delay/1

== system PvtSubSys_LSM/Subsystem/TargetLineCalc_20ms/TargetLineCalc/Subsystem3/Subsystem2/Subsystem6 ==
  u : Inport
  MATLAB Function14 : MATLAB Function  TreatAsAtomicUnit=on
  Unit Delay : UnitDelay  SampleTime=-1  HasFrameUpgradeWarning=on
  y : Outport
  wires:
  MATLAB Function14/2(i) -> Unit Delay/1
  u/1 -> MATLAB Function14/1(u)
  Unit Delay/1 -> MATLAB Function14/2(i_k)
  MATLAB Function14/1(y) -> y/1

== system PvtSubSys_LSM/Subsystem/TargetLineCalc_20ms/TargetLineCalc/Subsystem3/Subsystem2/Subsystem7 ==
  u : Inport
  MATLAB Function14 : MATLAB Function  TreatAsAtomicUnit=on
  Unit Delay : UnitDelay  SampleTime=-1  HasFrameUpgradeWarning=on
  y : Outport
  wires:
  MATLAB Function14/1(y) -> y/1
  Unit Delay/1 -> MATLAB Function14/2(i_k)
  u/1 -> MATLAB Function14/1(u)
  MATLAB Function14/2(i) -> Unit Delay/1

== system PvtSubSys_LSM/Subsystem/TargetLineCalc_20ms/TargetLineCalc/Subsystem3/Subsystem2/Subsystem8 ==
  u : Inport
  MATLAB Function14 : MATLAB Function  TreatAsAtomicUnit=on
  Unit Delay : UnitDelay  SampleTime=-1  HasFrameUpgradeWarning=on
  y : Outport
  wires:
  MATLAB Function14/2(i) -> Unit Delay/1
  u/1 -> MATLAB Function14/1(u)
  Unit Delay/1 -> MATLAB Function14/2(i_k)
  MATLAB Function14/1(y) -> y/1

== system PvtSubSys_LSM/Subsystem/TargetLineCalc_20ms/TargetLineCalc/Subsystem3/Subsystem2/Subsystem9 ==
  u : Inport
  MATLAB Function14 : MATLAB Function  TreatAsAtomicUnit=on
  Unit Delay : UnitDelay  SampleTime=-1  HasFrameUpgradeWarning=on
  y : Outport
  wires:
  MATLAB Function14/1(y) -> y/1
  Unit Delay/1 -> MATLAB Function14/2(i_k)
  u/1 -> MATLAB Function14/1(u)
  MATLAB Function14/2(i) -> Unit Delay/1

== matlab function PvtSubSys_LSM/Subsystem/TargetLineCalc_20ms/LHLine ==
  data: LH_Count input; LH1A0 input single size=1; LH1A1 input single size=1; LH1A2 input single size=1; LH1A3 input single size=1; LH1RaMin input single size=1; LH1RaMax input single size=1; LH1Conf output uint8 size=1; LH1Avail input uint8 size=1; LH1LineType input uint8 size=1; LH1DLType input uint8 size=1; LH1SideType input uint8 size=1; LH1Wid input single size=1; LH1Crossing input; LH1Confidence input; LH1_Color input; LH1DEType input; LH2A0 input single size=1; LH2A1 input single size=1; LH2A2 input single size=1; LH2A3 input single size=1; LH2RaMin input single size=1; LH2RaMax input single size=1; LH2Avail input uint8 size=1; LH2LineType input uint8 size=1; LH2DLType input uint8 size=1; LH2SideType input uint8 size=1; LH2Wid input single size=1; LH1C0 output single size=1; LH1C1 output single size=1; LH1C2 output single size=1; LH1C3 output single size=1; LH1DxMin output single size=1; LH1DxMax output single size=1; LH1Type output uint8 size=1; LH1DLM output uint8 size=1; LH1Width output single size=1; LH1Reliable output; LeftLaneChange output uint8 size=1; LH1Color output; LH1DECEL output; LH2Conf output uint8 size=1; LH2C0 output single size=1; LH2C1 output single size=1; LH2C2 output single size=1; LH2C3 output single size=1; LH2DxMin output single size=1; LH2DxMax output single size=1; LH2Type output uint8 size=1; LH2DLM output uint8 size=1; LH2Width output single size=1; LH2Reliable output; RightLaneChange output uint8 size=1; LH2Crossing input; LH2Confidence input; LH2_Color input; LH2Color output; LH2DEType input; LH2DECEL output
function [LH1Conf,LH1C0,LH1C1,LH1C2,LH1C3,LH1DxMin,LH1DxMax,LH1Type,LH1DLM,LH1Width,LH1Reliable,LeftLaneChange,LH1Color,LH1DECEL,...
    LH2Conf,LH2C0,LH2C1,LH2C2,LH2C3,LH2DxMin,LH2DxMax,LH2Type,LH2DLM,LH2Width,LH2Reliable,RightLaneChange,LH2Color,LH2DECEL]...
    = LH(LH_Count,LH1A0,LH1A1,LH1A2,LH1A3,LH1RaMin,LH1RaMax,LH1Avail,LH1LineType,LH1DLType,LH1SideType,LH1Wid,LH1Crossing,LH1Confidence,LH1_Color,LH1DEType,...
    LH2A0,LH2A1,LH2A2,LH2A3,LH2RaMin,LH2RaMax,LH2Avail,LH2LineType,LH2DLType,LH2SideType,LH2Wid,LH2Crossing,LH2Confidence,LH2_Color,LH2DEType)

LH1Conf = uint8(0);
LH1C0 = single(0);
LH1C1 = single(0);
LH1C2 = single(0);
LH1C3 = single(0);
LH1DxMin = single(0);
LH1DxMax = single(0);
LH1Type = uint8(0);
LH1DLM = uint8(0);
LH1Width = single(0);
LH1Reliable = single(0);
LeftLaneChange = uint8(0);
LH1Color = uint8(0);
LH1DECEL = uint8(0);

LH2Conf = uint8(0);
LH2C0 = single(0);
LH2C1 = single(0);
LH2C2 = single(0);
LH2C3 = single(0);
LH2DxMin = single(0);
LH2DxMax = single(0);
LH2Type = uint8(0);
LH2DLM = uint8(0);
LH2Width = single(0);
LH2Reliable = single(0);
RightLaneChange = uint8(0);
LH2Color = uint8(0);
LH2DECEL = uint8(0);


%%        自车道车道线预处理
if LH_Count >= 1                                       %车道线数量
    if LH1SideType==1                                  %左侧车道线
        LH1Conf = LH1Avail;
        LH1C0 = LH1A0;
        LH1C1 = LH1A1;
        LH1C2 = LH1A2;
        LH1C3 = LH1A3;
        LH1DxMin = LH1RaMin;
        LH1DxMax = LH1RaMax;
        LH1Type = LH1LineType;
        LH1DLM = LH1DLType;
        LH1Width = LH1Wid;
        LH1Reliable = LH1Confidence;
        LeftLaneChange = LH1Crossing;
        LH1Color = LH1_Color;
        LH1DECEL = LH1DEType;
    elseif LH1SideType==2                              %右侧车道线
        LH2Conf = LH1Avail;
        LH2C0 = LH1A0;
        LH2C1 = LH1A1;
        LH2C2 = LH1A2;
        LH2C3 = LH1A3;
        LH2DxMin = LH1RaMin;
        LH2DxMax = LH1RaMax;
        LH2Type = LH1LineType;
        LH2DLM = LH1DLType;
        LH2Width = LH1Wid;
        LH2Reliable = LH1Confidence;
        RightLaneChange = LH1Crossing;
        LH2Color = LH1_Color;
        LH2DECEL = LH1DEType;
    end
    if LH_Count >= 2
        if LH2SideType==1
            LH1Conf = LH2Avail;
            LH1C0 = LH2A0;
            LH1C1 = LH2A1;
            LH1C2 = LH2A2;
            LH1C3 = LH2A3;
            LH1DxMin = LH2RaMin;
            LH1DxMax = LH2RaMax;
            LH1Type = LH2LineType;
            LH1DLM = LH2DLType;
            LH1Width = LH2Wid;
            LH1Reliable = LH2Confidence;
            LeftLaneChange = LH2Crossing;
            LH1Color = LH2_Color;
            LH1DECEL = LH2DEType;
        elseif LH2SideType==2
            LH2Conf = LH2Avail;
            LH2C0 = LH2A0;
            LH2C1 = LH2A1;
            LH2C2 = LH2A2;
            LH2C3 = LH2A3;
            LH2DxMin = LH2RaMin;
            LH2DxMax = LH2RaMax;
            LH2Type = LH2LineType;
            LH2DLM = LH2DLType;
            LH2Width = LH2Wid;
            LH2Reliable = LH2Confidence;
            RightLaneChange = LH2Crossing;
            LH2Color = LH2_Color;
            LH2DECEL = LH2DEType;
        end
    end
end

== matlab function PvtSubSys_LSM/Subsystem/TargetLineCalc_20ms/LHLine1 ==
  data: LHA0 input single size=1; LHA1 input single size=1; LHA2 input single size=1; LHA3 input single size=1; LHRaMin input single size=1; LHRaMax input single size=1; LH_ELEM_Second_C0 input single size=1; LH_ELEM_Second_C1 input single size=1; LH_ELEM_Second_C2 input single size=1; LH_ELEM_Second_C3 input single size=1; LH_ELEM_Second_Start input single size=1; LH_ELEM_Second_End input single size=1; LHC0 output single size=1; LHC1 output single size=1; LHC2 output single size=1; LHC3 output single size=1; LHDxMin output single size=1; LHDxMax output single size=1
function [LHC0,LHC1,LHC2,LHC3,LHDxMin,LHDxMax]...
    = LH(LHA0,LHA1,LHA2,LHA3,LHRaMin,LHRaMax,...
    LH_ELEM_Second_C0,LH_ELEM_Second_C1,LH_ELEM_Second_C2,LH_ELEM_Second_C3,LH_ELEM_Second_Start,LH_ELEM_Second_End)

Second_Range = LH_ELEM_Second_End -LH_ELEM_Second_Start;

if Second_Range>0.5
%    [LineC3,LineC2,LineC1,LineC0,RangeMin,RangeMax]=CurveFitting(LH_ELEM_Second_C0,LH_ELEM_Second_C1,LH_ELEM_Second_C2,LH_ELEM_Second_C3,LH_ELEM_Second_Start,LH_ELEM0_Second_End,...
%   LHA0,LHA1,LHA2,LHA3,LHRaMin,LHRaMax,preDis);
%             LHC0 = LineC0;
%             LHC1 = LineC1;
%             LHC2 = LineC2;
%             LHC3 = LineC3;
%             LHDxMin = RangeMin;
%             LHDxMax = RangeMax;
    temp_x = [0.3*LHRaMax,0.5*LHRaMax,0.8*LHRaMax,LHRaMax+0.3*(LH_ELEM_Second_End-LH_ELEM_Second_Start),...
        LHRaMax+0.5*(LH_ELEM_Second_End-LH_ELEM_Second_Start),LHRaMax+0.8*(LH_ELEM_Second_End-LH_ELEM_Second_Start)];
  
        y1 = LHA0+LHA1*temp_x(1)+LHA2*temp_x(1)^2+LHA3*temp_x(1)^3;
        y2 = LHA0+LHA1*temp_x(2)+LHA2*temp_x(2)^2+LHA3*temp_x(2)^3;
        y3 = LHA0+LHA1*temp_x(3)+LHA2*temp_x(3)^2+LHA3*temp_x(3)^3;
        y4 = LH_ELEM_Second_C0+LH_ELEM_Second_C1*temp_x(4)+LH_ELEM_Second_C2*temp_x(4)^2+LH_ELEM_Second_C3*temp_x(4)^3;
        y5 = LH_ELEM_Second_C0+LH_ELEM_Second_C1*temp_x(5)+LH_ELEM_Second_C2*temp_x(5)^2+LH_ELEM_Second_C3*temp_x(5)^3;
        y6 = LH_ELEM_Second_C0+LH_ELEM_Second_C1*temp_x(6)+LH_ELEM_Second_C2*temp_x(6)^2+LH_ELEM_Second_C3*temp_x(6)^3;
    temp_y = [y1,y2,y3,y4,y5,y6];
    P = polyfit(temp_x,temp_y,2);
    LHC3 = single(0);
    LHC2 = P(1);
    LHC1 = P(2);
    LHC0 = P(3);
    Range=LH_ELEM_Second_End-LH_ELEM_Second_Start;
    if Range>0.5
        LHDxMin = LHRaMin;
        LHDxMax = LH_ELEM_Second_End;
    else
         LHDxMin = LHRaMin;
         LHDxMax = LHRaMax;
    end
else
    LHC0 = LHA0;
    LHC1 = LHA1;
    LHC2 = LHA2;
    LHC3 = LHA3;
    LHDxMin = LHRaMin;
    LHDxMax = LHRaMax;
end
end

%%


%% 
% function [LineC3,LineC2,LineC1,LineC0,RangeMin,RangeMax]=CurveFitting(Second_C0,Second_C1,Second_C2,Second_C3,Second_Start,Second_End,...
%     First_C0,First_C1,First_C2,First_C3,First_Start,First_Start_End,preDis)
% 
% temp_x = [0.4*preDis,0.8*preDis,preDis,1.2*preDis];
% if 0.4*preDis<Second_Start
%     y1 = First_C0+First_C1*temp_x(1)+First_C2*temp_x(1)^2+First_C3*temp_x(1)^3;
% else
%     y1 = Second_C0+Second_C1*temp_x(1)+Second_C2*temp_x(1)^2+Second_C3*temp_x(1)^3;
% end
% if 0.8*preDis<Second_Start
%     y2 = First_C0+First_C1*temp_x(2)+First_C2*temp_x(2)^2+First_C3*temp_x(2)^3;
% else
%     y2 = Second_C0+Second_C1*temp_x(2)+Second_C2*temp_x(2)^2+Second_C3*temp_x(2)^3;
% end
% 
% if preDis<Second_Start
%     y3 = First_C0+First_C1*temp_x(3)+First_C2*temp_x(3)^2+First_C3*temp_x(3)^3;
% else
%     y3 = Second_C0+Second_C1*temp_x(3)+Second_C2*temp_x(3)^2+Second_C3*temp_x(3)^3;
% end
% 
% if 1.2*preDis<Second_Start
%     y4 = First_C0+First_C1*temp_x(4)+First_C2*temp_x(4)^2+First_C3*temp_x(4)^3;
% else
%     y4 = Second_C0+Second_C1*temp_x(4)+Second_C2*temp_x(4)^2+Second_C3*temp_x(3)^3;
% end
% temp_y = [y1,y2,y3,y4];
% [LineC3,LineC2,LineC1,LineC0] = pl(temp_x,temp_y);
% 
% Range=Second_End-Second_Start;
% if Range>0.5
%     RangeMin = First_Start;
%     RangeMax = Second_End;
% else
%     RangeMin = First_Start;
%     RangeMax = First_Start_End;
% end  
% end

== matlab function PvtSubSys_LSM/Subsystem/TargetLineCalc_20ms/LHLine2 ==
  data: LHA0 input single size=1; LHA1 input single size=1; LHA2 input single size=1; LHA3 input single size=1; LHRaMin input single size=1; LHRaMax input single size=1; LH_ELEM_Second_C0 input single size=1; LH_ELEM_Second_C1 input single size=1; LH_ELEM_Second_C2 input single size=1; LH_ELEM_Second_C3 input single size=1; LH_ELEM_Second_Start input single size=1; LH_ELEM_Second_End input single size=1; LHC0 output single size=1; LHC1 output single size=1; LHC2 output single size=1; LHC3 output single size=1; LHDxMin output single size=1; LHDxMax output single size=1
function [LHC0,LHC1,LHC2,LHC3,LHDxMin,LHDxMax]...
    = LH(LHA0,LHA1,LHA2,LHA3,LHRaMin,LHRaMax,...
    LH_ELEM_Second_C0,LH_ELEM_Second_C1,LH_ELEM_Second_C2,LH_ELEM_Second_C3,LH_ELEM_Second_Start,LH_ELEM_Second_End)

Second_Range = LH_ELEM_Second_End -LH_ELEM_Second_Start;

if Second_Range>0.5
%    [LineC3,LineC2,LineC1,LineC0,RangeMin,RangeMax]=CurveFitting(LH_ELEM_Second_C0,LH_ELEM_Second_C1,LH_ELEM_Second_C2,LH_ELEM_Second_C3,LH_ELEM_Second_Start,LH_ELEM0_Second_End,...
%   LHA0,LHA1,LHA2,LHA3,LHRaMin,LHRaMax,preDis);
%             LHC0 = LineC0;
%             LHC1 = LineC1;
%             LHC2 = LineC2;
%             LHC3 = LineC3;
%             LHDxMin = RangeMin;
%             LHDxMax = RangeMax;
    temp_x = [0.3*LHRaMax,0.5*LHRaMax,0.8*LHRaMax,LHRaMax+0.3*(LH_ELEM_Second_End-LH_ELEM_Second_Start),...
        LHRaMax+0.5*(LH_ELEM_Second_End-LH_ELEM_Second_Start),LHRaMax+0.8*(LH_ELEM_Second_End-LH_ELEM_Second_Start)];
  
        y1 = LHA0+LHA1*temp_x(1)+LHA2*temp_x(1)^2+LHA3*temp_x(1)^3;
        y2 = LHA0+LHA1*temp_x(2)+LHA2*temp_x(2)^2+LHA3*temp_x(2)^3;
        y3 = LHA0+LHA1*temp_x(3)+LHA2*temp_x(3)^2+LHA3*temp_x(3)^3;
        y4 = LH_ELEM_Second_C0+LH_ELEM_Second_C1*temp_x(4)+LH_ELEM_Second_C2*temp_x(4)^2+LH_ELEM_Second_C3*temp_x(4)^3;
        y5 = LH_ELEM_Second_C0+LH_ELEM_Second_C1*temp_x(5)+LH_ELEM_Second_C2*temp_x(5)^2+LH_ELEM_Second_C3*temp_x(5)^3;
        y6 = LH_ELEM_Second_C0+LH_ELEM_Second_C1*temp_x(6)+LH_ELEM_Second_C2*temp_x(6)^2+LH_ELEM_Second_C3*temp_x(6)^3;
    temp_y = [y1,y2,y3,y4,y5,y6];
    P = polyfit(temp_x,temp_y,2);
    LHC3 = single(0);
    LHC2 = P(1);
    LHC1 = P(2);
    LHC0 = P(3);
    Range=LH_ELEM_Second_End-LH_ELEM_Second_Start;
    if Range>0.5
        LHDxMin = LHRaMin;
        LHDxMax = LH_ELEM_Second_End;
    else
         LHDxMin = LHRaMin;
         LHDxMax = LHRaMax;
    end
else
    LHC0 = LHA0;
    LHC1 = LHA1;
    LHC2 = LHA2;
    LHC3 = LHA3;
    LHDxMin = LHRaMin;
    LHDxMax = LHRaMax;
end
end

%%


%% 
% function [LineC3,LineC2,LineC1,LineC0,RangeMin,RangeMax]=CurveFitting(Second_C0,Second_C1,Second_C2,Second_C3,Second_Start,Second_End,...
%     First_C0,First_C1,First_C2,First_C3,First_Start,First_Start_End,preDis)
% 
% temp_x = [0.4*preDis,0.8*preDis,preDis,1.2*preDis];
% if 0.4*preDis<Second_Start
%     y1 = First_C0+First_C1*temp_x(1)+First_C2*temp_x(1)^2+First_C3*temp_x(1)^3;
% else
%     y1 = Second_C0+Second_C1*temp_x(1)+Second_C2*temp_x(1)^2+Second_C3*temp_x(1)^3;
% end
% if 0.8*preDis<Second_Start
%     y2 = First_C0+First_C1*temp_x(2)+First_C2*temp_x(2)^2+First_C3*temp_x(2)^3;
% else
%     y2 = Second_C0+Second_C1*temp_x(2)+Second_C2*temp_x(2)^2+Second_C3*temp_x(2)^3;
% end
% 
% if preDis<Second_Start
%     y3 = First_C0+First_C1*temp_x(3)+First_C2*temp_x(3)^2+First_C3*temp_x(3)^3;
% else
%     y3 = Second_C0+Second_C1*temp_x(3)+Second_C2*temp_x(3)^2+Second_C3*temp_x(3)^3;
% end
% 
% if 1.2*preDis<Second_Start
%     y4 = First_C0+First_C1*temp_x(4)+First_C2*temp_x(4)^2+First_C3*temp_x(4)^3;
% else
%     y4 = Second_C0+Second_C1*temp_x(4)+Second_C2*temp_x(4)^2+Second_C3*temp_x(3)^3;
% end
% temp_y = [y1,y2,y3,y4];
% [LineC3,LineC2,LineC1,LineC0] = pl(temp_x,temp_y);
% 
% Range=Second_End-Second_Start;
% if Range>0.5
%     RangeMin = First_Start;
%     RangeMax = Second_End;
% else
%     RangeMin = First_Start;
%     RangeMax = First_Start_End;
% end  
% end

== matlab function PvtSubSys_LSM/Subsystem/TargetLineCalc_20ms/LRELine ==
  data: LRE_Count input uint8 size=1; LRE1A0 input single size=1; LRE1A1 input single size=1; LRE1A2 input single size=1; LRE1A3 input single size=1; LRE1RaMin input single size=1; LRE1RaMax input single size=1; LRE1Conf output uint8 size=1; LRE1Avail input uint8 size=1; LRE1SideType input uint8 size=1; LRE1Confdience input; LRE2A0 input single size=1; LRE2A1 input single size=1; LRE2A2 input single size=1; LRE2A3 input single size=1; LRE2RaMin input single size=1; LRE2RaMax input single size=1; LRE2Avail input uint8 size=1; LRE2SideType input uint8 size=1; LRE1C0 output single size=1; LRE1C1 output single size=1; LRE1C2 output single size=1; LRE1C3 output single size=1; LRE1DxMin output single size=1; LRE1DxMax output single size=1; LRE1Reliable output; LRE2Conf output uint8 size=1; LRE2C0 output single size=1; LRE2C1 output single size=1; LRE2C2 output single size=1; LRE2C3 output single size=1; LRE2DxMin output single size=1; LRE2DxMax output single size=1; LRE2Confdience input; LRE2Reliable output
function [LRE1Conf,LRE1C0,LRE1C1,LRE1C2,LRE1C3,LRE1DxMin,LRE1DxMax,LRE1Reliable,...
    LRE2Conf,LRE2C0,LRE2C1,LRE2C2,LRE2C3,LRE2DxMin,LRE2DxMax,LRE2Reliable]...
    = LRE(LRE_Count,LRE1A0,LRE1A1,LRE1A2,LRE1A3,LRE1RaMin,LRE1RaMax,LRE1Avail,LRE1SideType,LRE1Confdience,...
    LRE2A0,LRE2A1,LRE2A2,LRE2A3,LRE2RaMin,LRE2RaMax,LRE2Avail,LRE2SideType,LRE2Confdience)

LRE1Conf = uint8(0);
LRE1C0 = single(0);
LRE1C1 = single(0);
LRE1C2 = single(0);
LRE1C3 = single(0);
LRE1DxMin = single(0);
LRE1DxMax = single(0);
LRE1Reliable = single(0);

LRE2Conf = uint8(0);
LRE2C0 = single(0);
LRE2C1 = single(0);
LRE2C2 = single(0);
LRE2C3 = single(0);
LRE2DxMin = single(0);
LRE2DxMax = single(0);
LRE2Reliable = single(0);

%%     边界线预处理
if LRE_Count == 2                                   %边界线数量
    if LRE1SideType==1                              %左侧边界线
        LRE1Conf = LRE1Avail;
        LRE1C0 = LRE1A0;
        LRE1C1 = LRE1A1;
        LRE1C2 = LRE1A2;
        LRE1C3 = LRE1A3;
        LRE1DxMin = LRE1RaMin;
        LRE1DxMax = LRE1RaMax;
        LRE1Reliable = LRE1Confdience;
    elseif LRE1SideType==2                           %右侧边界线
        LRE2Conf = LRE1Avail;
        LRE2C0 = LRE1A0;
        LRE2C1 = LRE1A1;
        LRE2C2 = LRE1A2;
        LRE2C3 = LRE1A3;
        LRE2DxMin = LRE1RaMin;
        LRE2DxMax = LRE1RaMax;
        LRE2Reliable = LRE1Confdience;
    end
    
    if LRE2SideType==1
        LRE1Conf = LRE2Avail;
        LRE1C0 = LRE2A0;
        LRE1C1 = LRE2A1;
        LRE1C2 = LRE2A2;
        LRE1C3 = LRE2A3;
        LRE1DxMin = LRE2RaMin;
        LRE1DxMax = LRE2RaMax;
        LRE1Reliable = LRE2Confdience;
    elseif LRE2SideType==2
        LRE2Conf = LRE2Avail;
        LRE2C0 = LRE2A0;
        LRE2C1 = LRE2A1;
        LRE2C2 = LRE2A2;
        LRE2C3 = LRE2A3;
        LRE2DxMin = LRE2RaMin;
        LRE2DxMax = LRE2RaMax;
        LRE2Reliable = LRE2Confdience;
    end
end

%%
if LRE_Count == 1
    if LRE1SideType==1
        LRE1Conf = LRE1Avail;
        LRE1C0 = LRE1A0;
        LRE1C1 = LRE1A1;
        LRE1C2 = LRE1A2;
        LRE1C3 = LRE1A3;
        LRE1DxMin = LRE1RaMin;
        LRE1DxMax = LRE1RaMax;
        LRE1Reliable = LRE1Confdience;
    elseif LRE1SideType==2
        LRE2Conf = LRE1Avail;
        LRE2C0 = LRE1A0;
        LRE2C1 = LRE1A1;
        LRE2C2 = LRE1A2;
        LRE2C3 = LRE1A3;
        LRE2DxMin = LRE1RaMin;
        LRE2DxMax = LRE1RaMax;
        LRE2Reliable = LRE1Confdience;
    end
end

== matlab function PvtSubSys_LSM/Subsystem/TargetLineCalc_20ms/MATLAB Function ==
  data: LA_Sync_ID input uint8 size=1; y output boolean size=1; LA_Update input boolean size=1; LH_Sync_ID input uint8 size=1; LH_Upadate input boolean size=1
function y = fcn(LA_Sync_ID,LA_Update,LH_Sync_ID,LH_Upadate)
if (LA_Sync_ID==LH_Sync_ID) && (LA_Update==true||LH_Upadate==true)
    y = true;
else
    y = false;
end
